simulink model "msk"  (R2020a)
settings: Solver=VariableStepAuto  StartTime=0.0  StopTime=10.0  RelTol=1e-3
libraries: commdigbbndcpm2 x2, commchan3 x1, commrandsrc3 x1
settings Model: Creator=uzend  LastModifiedBy=demid

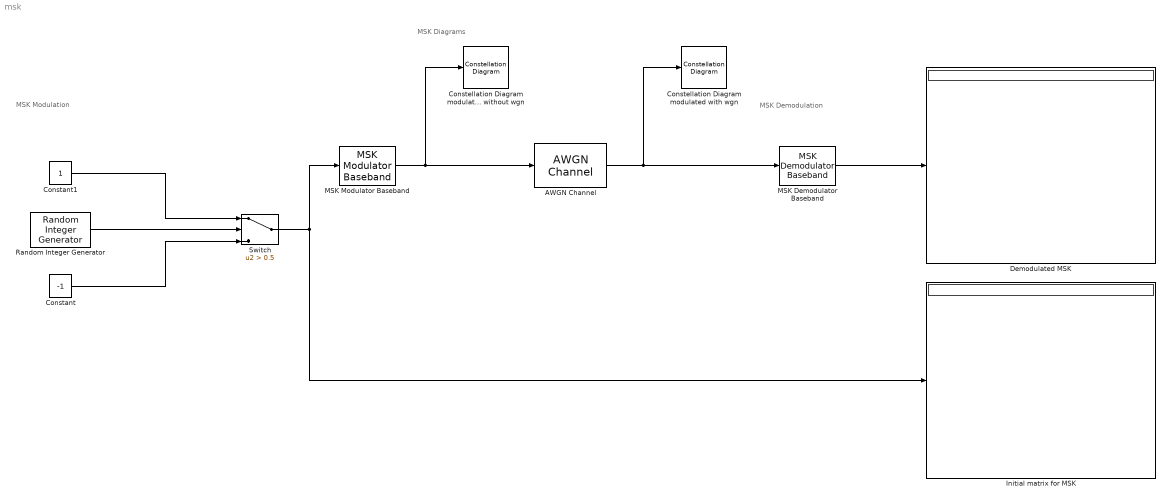
== system msk ==
  note: MSK Demodulation
  note: MSK Diagrams
  note: MSK Modulation
  AWGN Channel : commchan3/AWGN Channel  InputProcessing=Columns as channels (frame based)  seed=67  noiseMode="Signal to noise ratio  (Eb/No)"  EbNodB=35  EsNodB=10  SNRdB=10  bitsPerSym=1  Ps=1  Tsym=1  variance=1
  Constant : Constant  Value=-1
  Constant1 : Constant
  Constellation Diagram modulated with wgn : ConstellationDiagram
  Constellation Diagram modulated without wgn : ConstellationDiagram
  Demodulated MSK : Display
  Initial matrix for MSK : Display
  MSK Demodulator Baseband : commdigbbndcpm2/MSK Demodulator Baseband  outputType=Integer  phaseOffset=0  samplesPerSymbol=8  RateOptions=Enforce single-rate processing  traceBack=16  outDType=double
      settings: SourceProductBaseCode=CM
  MSK Modulator Baseband : commdigbbndcpm2/MSK Modulator Baseband  inputType=Integer  phaseOffset=0  samplesPerSymbol=8  RateOptions=Enforce single-rate processing  outDataType=double
      settings: SourceProductBaseCode=CM
  Random Integer Generator : commrandsrc3/Random Integer Generator  SetSize=2  SeedSource=Auto  Seed=0  SampleTime=1  SamplesPerFrame=100  OutputDataType=double  SimulateUsing=Interpreted execution
  Switch : Switch  Criteria=u2 > Threshold  Threshold=0.5
  wires:
  MSK Modulator Baseband/1 -> AWGN Channel/1, Constellation Diagram modulated without wgn/1
  AWGN Channel/1 -> MSK Demodulator Baseband/1, Constellation Diagram modulated with wgn/1
  MSK Demodulator Baseband/1 -> Demodulated MSK/1
  Switch/1 -> Initial matrix for MSK/1, MSK Modulator Baseband/1
  Random Integer Generator/1 -> Switch/2
  Constant/1 -> Switch/3
  Constant1/1 -> Switch/1
